simulink model "simulink_model"  (R2023a)
settings: Solver=VariableStepAuto  StartTime=0.0  StopTime=1  RelTol=1e-3
undefined symbols (not defined in the file or in its folder): center, scale
libraries: deeplib x1, matrix_library x1
settings Model: Creator=orfea  LastModifiedBy=orfea
settings OptimizationCC: ZeroExternalMemoryAtStartup=off  ZeroInternalMemoryAtStartup=off
settings HardwareCC: ProdHWDeviceType=AMD->x86-64 (Windows64)
settings RTWCC: TargetLang=C++  CheckMdlBeforeBuild=Warning
settings GRTTargetCC: TargetLangStandard=C++11 (ISO)  CodeInterfacePackaging=C++ class

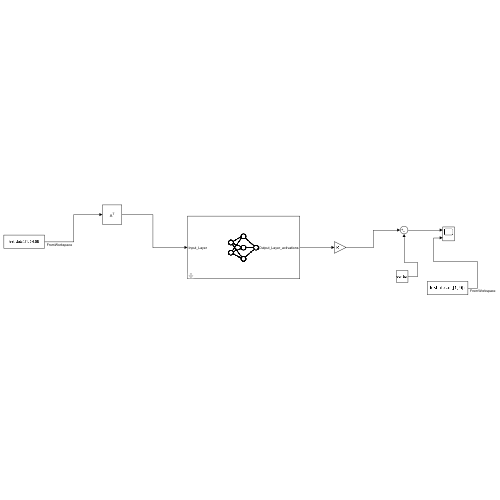
[thumbnail: Simulink's stored preview of the top-level diagram]
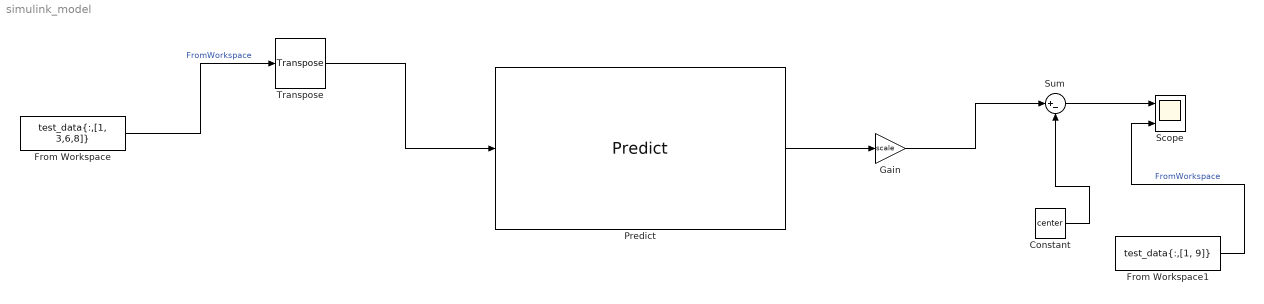
== system simulink_model ==
  Constant : Constant  Value=center  VectorParams1D=off
  From Workspace : FromWorkspace  VariableName=test_data{:,[1, 3,6,8]}  OutDataTypeStr=double  SampleTime=0.01
  From Workspace1 : FromWorkspace  VariableName=test_data{:,[1, 9]}  OutDataTypeStr=double  SampleTime=0.01
  Gain : Gain  Gain=scale
  Predict : deeplib/Predict  Network=Network from MAT-file  NetworkFunction=squeezenet  NetworkFilePath=D:\Orfeas\PhD\Teaching_Assistant\Advanced_Automated_Systems\Advanced-ACS\Spring2024\Lectures\models\net_checkpoint__360__2024_05_17__06_42_47.mat  MiniBatchSize=128  InputDataFormats={'',''}  Predictions=off  Activations={'Output_Layer'}  ForceInterpretedSim=off  EnableDLNetwork=on
  Scope : Scope  NumInputPorts=2
  Sum : Sum  Inputs=|+-
  Transpose : matrix_library/Transpose
  wires:
  From Workspace/1 -> Transpose/1  "FromWorkspace"
  Predict/1 -> Gain/1
  Transpose/1 -> Predict/1
  Gain/1 -> Sum/1
  Constant/1 -> Sum/2
  Sum/1 -> Scope/1
  From Workspace1/1 -> Scope/2  "FromWorkspace"
